simulink model "UAM_GuidanceAndNavigation"  (R2024b)
settings: Solver=FixedStepAuto  StartTime=0.0  StopTime=10.0  RelTol=1e-3
undefined symbols (not defined in the file): Earth, WGS84
libraries: simulink x2, robotcorelib x2, uavalgslib x1, mspfiltlib x1, simulink_extras x1, aerolibtransform2 x1
settings Model: DataDictionary=UAM_data.sldd  Creator=admin  LastModifiedBy=admin
settings OptimizationCC: DefaultParameterBehavior=Inlined  EnhancedBackFolding=on  PassReuseOutputArgsAs=Individual arguments  ZeroExternalMemoryAtStartup=off  ZeroInternalMemoryAtStartup=off  OptimizeBlockOrder=speed  DifferentSizesBufferReuse=on  OptimizationCustomize=off  EfficientTunableParamExpr=on
settings DebuggingCC: ParameterTunabilityLossMsg=error
settings HardwareCC: ProdBitPerLong=64  ProdLargestAtomicInteger=LongLong  ProdLargestAtomicFloat=Double  ProdLongLongMode=on  ProdHWDeviceType=ARM Compatible->ARM Cortex-A (64-bit)
settings SFSimCC: MATLABDynamicMemAlloc=off
settings RTWCC: Description=Embedded Coder  SystemTargetFile=ert.tlc  TemplateMakefile=ert_default_tmf  Toolchain=Linaro AArch64 Linux v6.3.1
settings CodeAppCC: ForceParamTrailComments=on  IgnoreCustomStorageClasses=off  OperatorAnnotations=on  SimulinkDataObjDesc=on  SFDataObjDesc=on  CustomSymbolStrGlobalVar=GUID_$N$M  CustomSymbolStrType=GUID_$N$M_T  CustomSymbolStrField=GUID_$N$M  CustomSymbolStrFcn=GUID_$N$M$F  CustomSymbolStrBlkIO=GUID_rtb_$N$M  CustomSymbolStrTmpVar=GUID_tmp_$N$M  CustomSymbolStrMacro=GUID_$N$M_MACRO  InsertBlockDesc=on
settings ERTTargetCC: TargetLangStandard=C99 (ISO)  GenerateSampleERTMain=on  ERTCustomFileTemplate=example_file_process.tlc

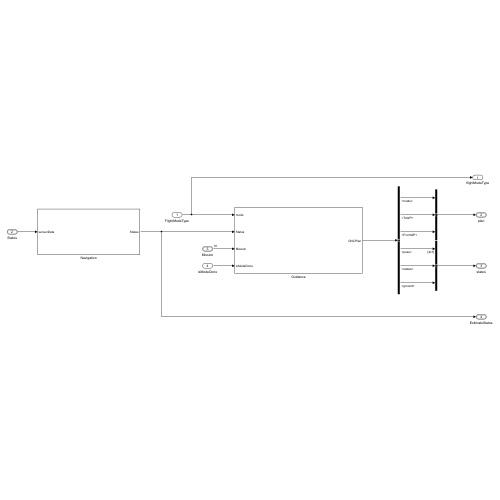
[thumbnail: Simulink's stored preview of the top-level diagram]
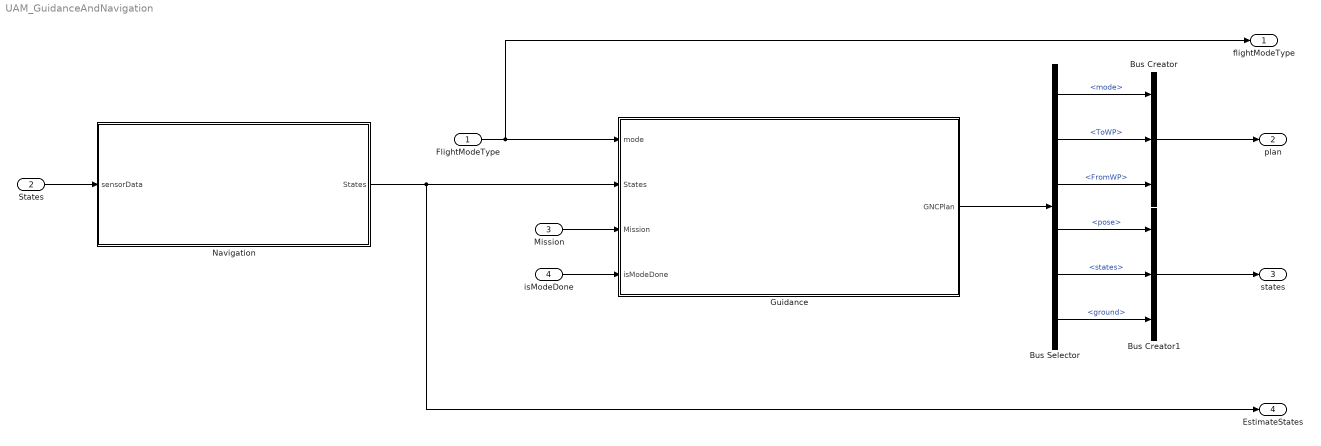
== system UAM_GuidanceAndNavigation ==
  FlightModeType : Inport  OutDataTypeStr=Enum: FlightModeType
  States : Inport  Port=2  OutDataTypeStr=Bus: sensorData
  Mission : Inport  Port=3  OutDataTypeStr=Bus: UAVPathManagerBus  PortDimensions=10  BusOutputAsStruct=on
  isModeDone : Inport  Port=4  OutDataTypeStr=uint8
  Bus Creator : BusCreator  Inputs=3  OutDataTypeStr=Bus: plan
      settings: InheritFromInputs=off
  Bus Creator1 : BusCreator  Inputs=3  OutDataTypeStr=Bus: states
      settings: InheritFromInputs=off
  Bus Selector : BusSelector  OutputSignals=mode,ToWP,FromWP,pose,states,ground
  Guidance : Subsystem
  Navigation : Subsystem
  flightModeType : Outport
  plan : Outport  Port=2  OutDataTypeStr=Bus: plan
  states : Outport  Port=3  OutDataTypeStr=Bus: states
  EstimateStates : Outport  Port=4  OutDataTypeStr=Bus: StateBus
  wires:
  Navigation/1(States) -> EstimateStates/1, Guidance/2(States)
  States/1 -> Navigation/1(sensorData)
  isModeDone/1 -> Guidance/4(isModeDone)
  FlightModeType/1 -> Guidance/1(mode), flightModeType/1
  Bus Creator1/1 -> states/1
  Bus Creator/1 -> plan/1
  Guidance/1(GNCPlan) -> Bus Selector/1
  Bus Selector/1 -> Bus Creator/1  "<mode>"
  Bus Selector/3 -> Bus Creator/3  "<FromWP>"
  Bus Selector/4 -> Bus Creator1/1  "<pose>"
  Bus Selector/5 -> Bus Creator1/2  "<states>"
  Bus Selector/6 -> Bus Creator1/3  "<ground>"
  Bus Selector/2 -> Bus Creator/2  "<ToWP>"
  Mission/1 -> Guidance/3(Mission)

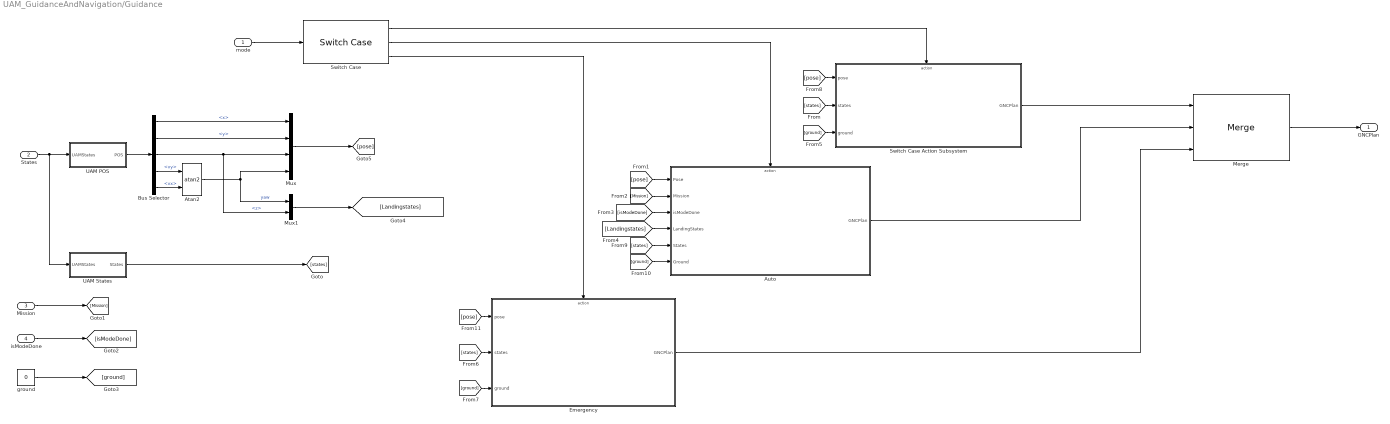
== system UAM_GuidanceAndNavigation/Guidance ==
  mode : Inport
  States : Inport  Port=2
  Mission : Inport  Port=3  OutDataTypeStr=Bus: UAVPathManagerBus
  isModeDone : Inport  Port=4
  Atan2 : Trigonometry  Operator=atan2
  Auto : Subsystem  TreatAsAtomicUnit=on
  Bus Selector : BusSelector  OutputSignals=x,y,z,vy,vx
  Emergency : Subsystem  TreatAsAtomicUnit=on
  Merge : Merge  Inputs=3
  Mux : Mux
  Mux1 : Mux  Inputs=2
  Switch Case : SwitchCase  CaseConditions={FlightModeType.Manual, FlightModeType.Auto, FlightModeType.Emergecny}  ShowDefaultCase=off
  Switch Case Action Subsystem : Subsystem  TreatAsAtomicUnit=on
  UAM POS : Subsystem
  UAM States : Subsystem
  ground : Constant  Value=0
  GNCPlan : Outport  OutDataTypeStr=Bus: GNCplan
  wires:
  mode/1 -> Switch Case/1
  [pose] -> Emergency/1(pose)
  UAM POS/1(POS) -> Bus Selector/1
  [ground] -> Auto/6(Ground)
  [states] -> Switch Case Action Subsystem/2(states)
  Bus Selector/1 -> Mux/1  "<x>"
  Mission/1 -> [Mission]
  [pose] -> Auto/1(Pose)
  [states] -> Emergency/2(states)
  [isModeDone] -> Auto/3(isModeDone)
  Emergency/1(GNCPlan) -> Merge/3
  [ground] -> Switch Case Action Subsystem/3(ground)
  Auto/1(GNCPlan) -> Merge/2
  [ground] -> Emergency/3(ground)
  Switch Case/1 -> Switch Case Action Subsystem/Action
  Bus Selector/2 -> Mux/2  "<y>"
  [Mission] -> Auto/2(Mission)
  Switch Case Action Subsystem/1(GNCPlan) -> Merge/1
  Atan2/1 -> Mux1/1, Mux/4  "yaw"
  ground/1 -> [ground]
  Mux/1 -> [pose]
  Merge/1 -> GNCPlan/1
  Switch Case/3 -> Emergency/Action
  [Landingstates] -> Auto/4(LandingStates)
  isModeDone/1 -> [isModeDone]
  [states] -> Auto/5(States)
  Bus Selector/3 -> Mux1/2, Mux/3  "<z>"
  UAM States/1(States) -> [states]
  [pose] -> Switch Case Action Subsystem/1(pose)
  Switch Case/2 -> Auto/Action
  Mux1/1 -> [Landingstates]
  States/1 -> UAM States/1(UAMStates), UAM POS/1(UAMStates)
  Bus Selector/4 -> Atan2/1  "<vy>"
  Bus Selector/5 -> Atan2/2  "<vx>"

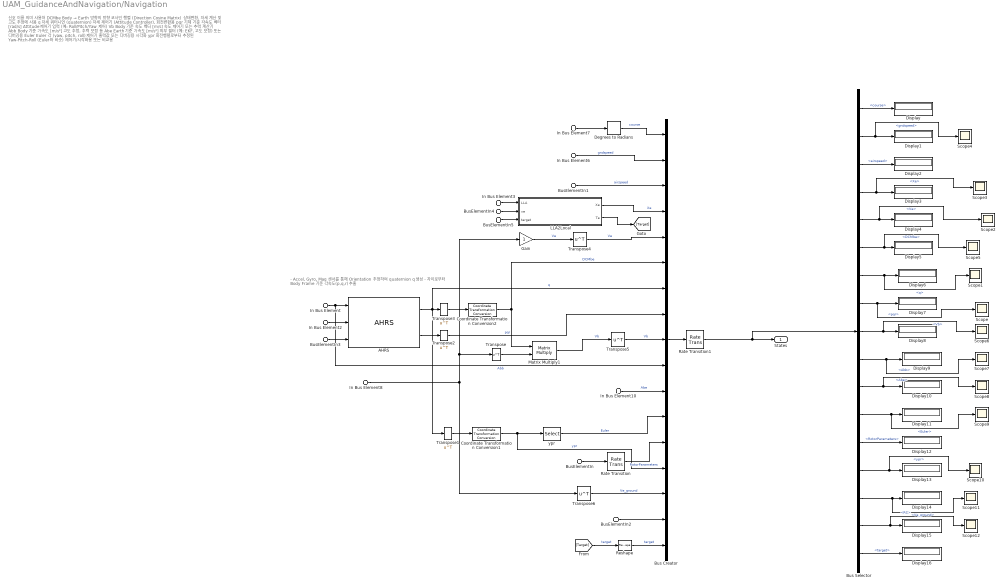
== system UAM_GuidanceAndNavigation/Navigation ==
  note: 신호 이름
      | 의미
      | 사용처
      |
      | DCMbe
      | Body → Earth 방향의 방향 코사인 행렬 (Direction Cosine Matrix)
      | 상태변환, 자세 계산 및 고도 추정에 사용
      |
      | q
      | 자세 쿼터니언 (quaternion)
      | 자세 제어기 (Attitude Controller), 회전변환용
      |
      | pqr
      | 기체 기준 각속도 벡터 [rad/s]
      | Attitude 제어기 입력 (예: Roll/Pitch/Yaw 제어)
      |
      | Vb
      | Body 기준 속도 벡터 [m/s]
      | 속도 제어기 또는 추력 계산기
      |
      | Abb
      | Body 기준 가속도 [m/s²]
      | 고도 추정, 추력 보정 등
      |
      | Abe
      | Earth 기준 가속도 [m/s²]
      | 외부 필터 (예: EKF, 고도 보정) 또는 디버깅용
      |
      | Euler
      | Euler 각 (yaw, pitch, roll)
      | 제어기 출력값 또는 디버깅용 시각화
      |
      | ypr
      | 회전행렬로부터 추정된 Yaw-Pitch-Roll (Euler와 비슷)
      | 제어기/시각화용 또는 비교용
  note: - Accel, Gyro, Mag 센서를 통해 Orientation 추정하여 quaternion q 생성
      | - 자이로부터 Body Frame 기준 각속도(p,q,r) 추출
  In Bus Element : Inport  PortName=sensorData  Element=Abb
  In Bus Element2 : Inport  PortName=sensorData  Element=Gyro
  In Bus Element3 : Inport  PortName=sensorData  Element=LLA
  In Bus Element6 : Inport  PortName=sensorData  Element=gndspeed
  In Bus Element7 : Inport  PortName=sensorData  Element=GPSCourse
  In Bus Element8 : Inport  PortName=sensorData  Element=GPSVelocity
  In Bus Element10 : Inport  PortName=sensorData  Element=Abe
  BusElementIn : Inport  PortName=sensorData  Element=RotorParameters
  BusElementIn1 : Inport  PortName=sensorData  Element=airspeed
  BusElementIn2 : Inport  PortName=sensorData  Element=RC
  BusElementIn5 : Inport  PortName=sensorData  Element=target
  BusElementIn3 : Inport  PortName=sensorData  Element=Mag
  BusElementIn4 : Inport  PortName=sensorData  Element=arming
  AHRS : mspfiltlib/AHRS  DispRefFrame=NED  DecimationFactor=1  InitialProcessNoise=ahrsfilter.defaultProcessNoise  OrientationFormat=quaternion  SimulateUsing=Interpreted execution  AccelerometerNoise=0.0001924722  GyroscopeNoise=9.1385e-5  MagnetometerNoise=0.1  GyroscopeDriftNoise=3.0462e-13  LinearAccelerationNoise=0.0096236100000000012  MagneticDisturbanceNoise=0.5  LinearAccelerationDecayFactor=0.5  MagneticDisturbanceDecayFactor=0.5  ExpectedMagneticFieldStrength=50
  Bus Creator : BusCreator  Inputs=17  OutDataTypeStr=Bus: StateBus
  Bus Selector : BusSelector  OutputSignals=course,gndspeed,airspeed,Xe,Ve,DCMbe,q,pqr,Vb,Abb,Abe,Euler,RotorParameters,ypr,Ve_ground,RC,target
  Coordinate Transformation Conversion1 : robotcorelib/Coordinate Transformation Conversion  InputRepresentation=Quaternion  InputEulerSequence=ZYX  ShowTrVecInputPort=on  OutputRepresentation=Euler Angles  OutputEulerSequence=ZYX  ShowTrVecOutputPort=on  SimulateUsing=Interpreted execution
  Coordinate Transformation Conversion2 : robotcorelib/Coordinate Transformation Conversion  InputRepresentation=Quaternion  InputEulerSequence=ZYX  ShowTrVecInputPort=on  OutputRepresentation=Rotation Matrix  OutputEulerSequence=ZYX  ShowTrVecOutputPort=on  SimulateUsing=Interpreted execution
  Degrees to Radians : simulink_extras/Transformations/Degrees to Radians
  Display{,1..16} (17 alike) : Display
  Gain : Gain
  LLA2Local : Subsystem
  Matrix Multiply1 : Product  Multiplication=Matrix(*)
  Rate Transition : RateTransition  OutPortSampleTime=0.001
  Rate Transition1 : RateTransition
  Reshape : Reshape  OutputDimensionality=Customize  OutputDimensions=[1 3]
  Scope{,1..12} (13 alike) : Scope
  Transpose{,1..6} (7 alike) : Math  Operator=transpose
  ypr : Selector  InputPortWidth=3  IndexOptions=Index vector (dialog)  Indices=[3 2 1]  OutputSizes=1
  States : Outport  OutDataTypeStr=Bus: StateBus
  wires:
  Transpose6/1 -> Bus Creator/15  "Ve_ground"
  In Bus Element/1 -> AHRS/1, Bus Creator/10  "Abb"
  ypr/1 -> Bus Creator/12  "Euler"
  Gain/1 -> Transpose4/1  "Ve"
  Transpose/1 -> Matrix Multiply1/2
  LLA2Local/1(Xe) -> Bus Creator/4  "Xe"
  Matrix Multiply1/1 -> Transpose5/1  "Vb"
  In Bus Element8/1 -> Gain/1, Transpose/1, Transpose6/1
  In Bus Element7/1 -> Degrees to Radians/1
  Rate Transition1/1 -> Bus Selector/1, States/1
  In Bus Element6/1 -> Bus Creator/2  "gndspeed"
  Coordinate Transformation Conversion2/1 -> Bus Creator/6, Matrix Multiply1/1  "DCMbe"
  Transpose5/1 -> Bus Creator/9  "Vb"
  Transpose2/1 -> Bus Creator/8  "pqr"
  Coordinate Transformation Conversion1/1 -> Bus Creator/14, ypr/1  "ypr"
  In Bus Element10/1 -> Bus Creator/11  "Abe"
  Bus Creator/1 -> Rate Transition1/1
  Rate Transition/1 -> Bus Creator/13  "RotorParameters"
  Degrees to Radians/1 -> Bus Creator/1  "course"
  Transpose4/1 -> Bus Creator/5  "Ve"
  In Bus Element3/1 -> LLA2Local/1(LLA)
  BusElementIn/1 -> Rate Transition/1
  BusElementIn1/1 -> Bus Creator/3  "airspeed"
  BusElementIn2/1 -> Bus Creator/16
  Transpose1/1 -> Coordinate Transformation Conversion1/1
  Transpose3/1 -> Coordinate Transformation Conversion2/1
  LLA2Local/2(Te) -> [Target]
  [Target] -> Reshape/1  "target"
  BusElementIn5/1 -> LLA2Local/3(target)
  Reshape/1 -> Bus Creator/17  "target"
  In Bus Element2/1 -> AHRS/2
  BusElementIn3/1 -> AHRS/3
  AHRS/1 -> Transpose3/1, Transpose1/1, Bus Creator/7  "q"
  AHRS/2 -> Transpose2/1
  BusElementIn4/1 -> LLA2Local/2(ve)
  Bus Selector/1 -> Display/1  "<course>"
  Bus Selector/2 -> Scope4/1, Display1/1  "<gndspeed>"
  Bus Selector/3 -> Display2/1  "<airspeed>"
  Bus Selector/4 -> Scope3/1, Display3/1  "<Xe>"
  Bus Selector/5 -> Scope2/1, Display4/1  "<Ve>"
  Bus Selector/6 -> Scope5/1, Display5/1  "<DCMbe>"
  Bus Selector/7 -> Scope1/1, Display6/1  "<q>"
  Bus Selector/8 -> Scope/1, Display7/1  "<pqr>"
  Bus Selector/9 -> Scope6/1, Display8/1  "<Vb>"
  Bus Selector/10 -> Scope7/1, Display9/1  "<Abb>"
  Bus Selector/11 -> Scope8/1, Display10/1  "<Abe>"
  Bus Selector/12 -> Scope9/1, Display11/1  "<Euler>"
  Bus Selector/13 -> Display12/1  "<RotorParameters>"
  Bus Selector/14 -> Scope10/1, Display13/1  "<ypr>"
  Bus Selector/15 -> Scope11/1, Display14/1  "<Ve_ground>"
  Bus Selector/16 -> Scope12/1, Display15/1  "<RC>"
  Bus Selector/17 -> Display16/1  "<target>"

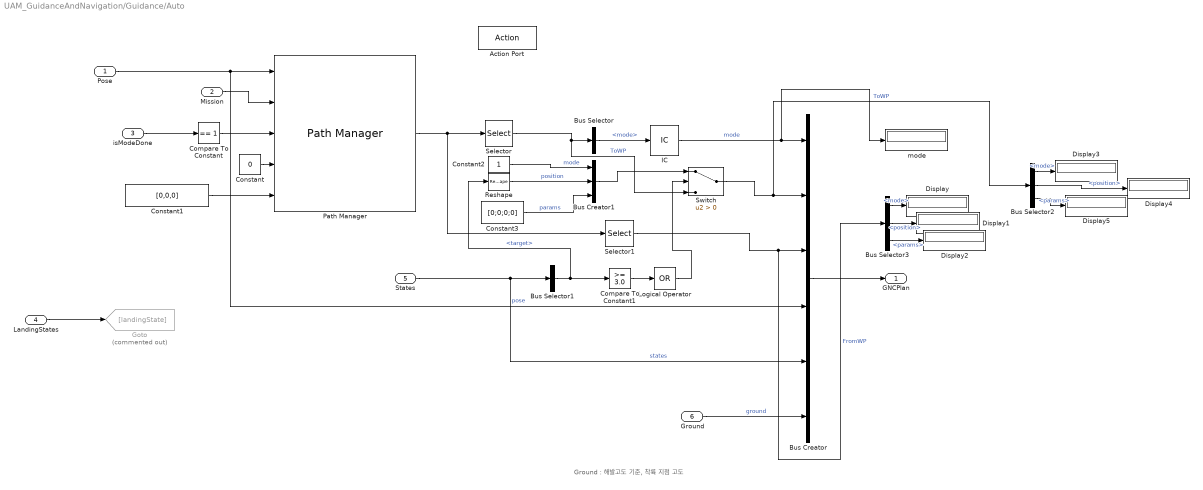
== system UAM_GuidanceAndNavigation/Guidance/Auto ==
  note: Ground : 해발고도 기준, 착륙 지점 고도
  Pose : Inport
  Mission : Inport  Port=2  OutDataTypeStr=Bus: UAVPathManagerBus
  isModeDone : Inport  Port=3
  LandingStates : Inport  Port=4
  States : Inport  Port=5
  Ground : Inport  Port=6
  Action Port : ActionPort  ActionPortLabel=case [ Auto ]:
  Bus Creator : BusCreator  Inputs=6  OutDataTypeStr=Bus: GNCplan
  Bus Creator1 : BusCreator  Inputs=3  OutDataTypeStr=Bus: UAVPathManagerBus  NonVirtualBus=on
  Bus Selector : BusSelector  OutputSignals=mode
  Bus Selector1 : BusSelector  OutputSignals=target
  Bus Selector2 : BusSelector  OutputSignals=mode,position,params
  Bus Selector3 : BusSelector  OutputSignals=mode,position,params
  Compare To Constant : simulink/Logic and Bit Operations/Compare To Constant  relop===  const=1  OutDataTypeStr=boolean
  Compare To Constant1 : simulink/Logic and Bit Operations/Compare To Constant  relop=>=  const=3.0  OutDataTypeStr=boolean
  Constant : Constant  Value=0  OutDataTypeStr=uint8
  Constant1 : Constant  Value=[0,0,0]  OutDataTypeStr=double
  Constant2 : Constant  OutDataTypeStr=uint8
  Constant3 : Constant  Value=[0;0;0;0]
  Display{,1..5} (6 alike) : Display
  Goto : Goto  Commented=on  GotoTag=landingState
  IC : InitialCondition
  Logical Operator : Logic  Operator=OR  Inputs=1  AllPortsSameDT=off  OutDataTypeStr=boolean
  Path Manager : uavalgslib/Path Manager  UAVType=multirotor  LoiterRadius=25  dataType=double  inputBusName='UAVPathManagerBus'  SimulateUsing=Code generation
  Reshape : Reshape  OutputDimensionality=Customize  OutputDimensions=[3 1]
  Selector : Selector  InputPortWidth=2  IndexOptions=Index vector (dialog)  Indices=1  OutputSizes=1
  Selector1 : Selector  InputPortWidth=2  IndexOptions=Index vector (dialog)  Indices=2  OutputSizes=1
  Switch : Switch  Criteria=u2 > Threshold  SaturateOnIntegerOverflow=off  InputSameDT=off
  mode : Display
  GNCPlan : Outport  OutDataTypeStr=Bus: GNCplan
  wires:
  IC/1 -> mode/1, Bus Creator/1  "mode"
  Ground/1 -> Bus Creator/6  "ground"
  Selector1/1 -> Bus Selector3/1, Bus Creator/3  "FromWP"
  States/1 -> Bus Selector1/1, Bus Creator/5  "states"
  Bus Creator/1 -> GNCPlan/1
  Selector/1 -> Bus Selector/1, Switch/3  "ToWP"
  Path Manager/1 -> Selector/1, Selector1/1
  Constant/1 -> Path Manager/4
  Constant1/1 -> Path Manager/5
  Pose/1 -> Bus Creator/4, Path Manager/1  "pose"
  LandingStates/1 -> Goto/1
  Compare To Constant/1 -> Path Manager/3
  isModeDone/1 -> Compare To Constant/1
  Bus Selector/1 -> IC/1  "<mode>"
  Mission/1 -> Path Manager/2
  Bus Selector1/1 -> Reshape/1, Compare To Constant1/1  "<target>"
  Compare To Constant1/1 -> Logical Operator/1
  Logical Operator/1 -> Switch/2
  Switch/1 -> Bus Selector2/1, Bus Creator/2  "ToWP"
  Constant2/1 -> Bus Creator1/1  "mode"
  Constant3/1 -> Bus Creator1/3  "params"
  Reshape/1 -> Bus Creator1/2  "position"
  Bus Creator1/1 -> Switch/1
  Bus Selector3/1 -> Display/1  "<mode>"
  Bus Selector3/2 -> Display1/1  "<position>"
  Bus Selector3/3 -> Display2/1  "<params>"
  Bus Selector2/1 -> Display3/1  "<mode>"
  Bus Selector2/2 -> Display4/1  "<position>"
  Bus Selector2/3 -> Display5/1  "<params>"

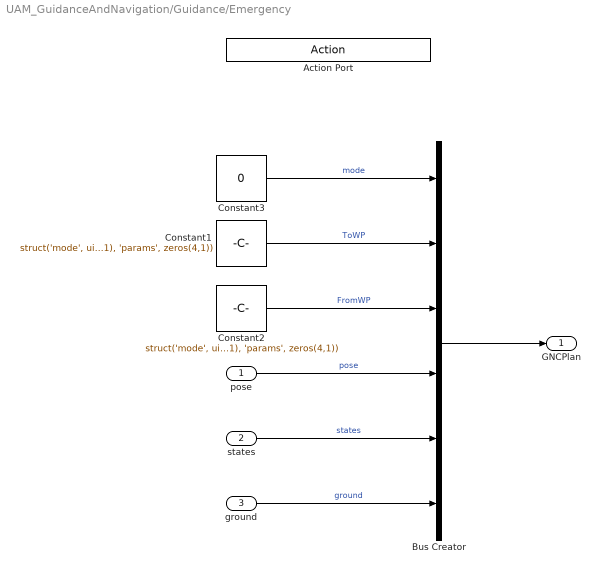
== system UAM_GuidanceAndNavigation/Guidance/Emergency ==
  pose : Inport
  states : Inport  Port=2
  ground : Inport  Port=3
  Action Port : ActionPort  ActionPortLabel=case [ Emergecny ]:
  Bus Creator : BusCreator  Inputs=6  OutDataTypeStr=Bus: GNCplan
  Constant1 : Constant  Value=struct('mode', uint8(0), 'position', zeros(3,1), 'params', zeros(4,1))  OutDataTypeStr=Bus: UAVPathManagerBus
  Constant2 : Constant  Value=struct('mode', uint8(0), 'position', zeros(3,1), 'params', zeros(4,1))  OutDataTypeStr=Bus: UAVPathManagerBus
  Constant3 : Constant  Value=0  OutDataTypeStr=uint8
  GNCPlan : Outport  OutDataTypeStr=Bus: GNCplan
  wires:
  pose/1 -> Bus Creator/4  "pose"
  Bus Creator/1 -> GNCPlan/1
  Constant1/1 -> Bus Creator/2  "ToWP"
  Constant2/1 -> Bus Creator/3  "FromWP"
  ground/1 -> Bus Creator/6  "ground"
  states/1 -> Bus Creator/5  "states"
  Constant3/1 -> Bus Creator/1  "mode"

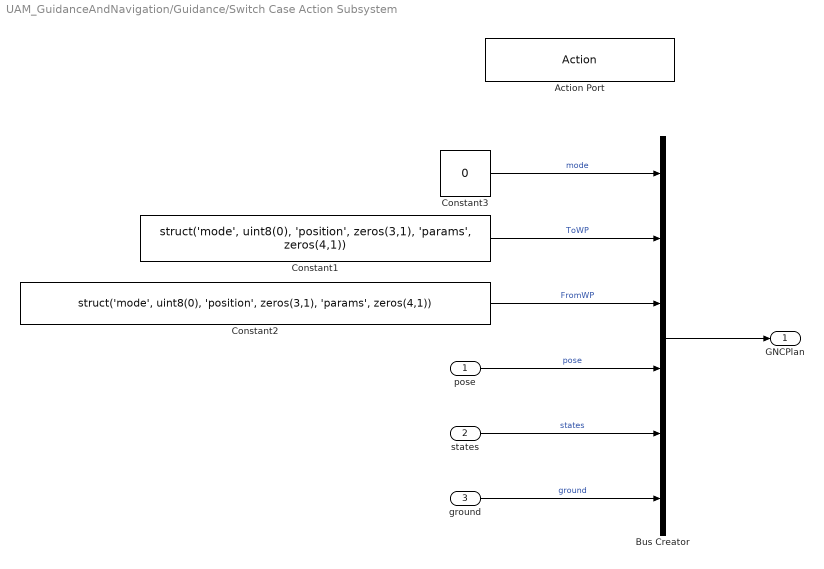
== system UAM_GuidanceAndNavigation/Guidance/Switch Case Action Subsystem ==
  pose : Inport
  states : Inport  Port=2
  ground : Inport  Port=3
  Action Port : ActionPort  ActionPortLabel=case [ Manual ]:
  Bus Creator : BusCreator  Inputs=6  OutDataTypeStr=Bus: GNCplan
  Constant1 : Constant  Value=struct('mode', uint8(0), 'position', zeros(3,1), 'params', zeros(4,1))  OutDataTypeStr=Bus: UAVPathManagerBus
  Constant2 : Constant  Value=struct('mode', uint8(0), 'position', zeros(3,1), 'params', zeros(4,1))  OutDataTypeStr=Bus: UAVPathManagerBus
  Constant3 : Constant  Value=0  OutDataTypeStr=uint8
  GNCPlan : Outport  OutDataTypeStr=Bus: GNCplan
  wires:
  Bus Creator/1 -> GNCPlan/1
  Constant3/1 -> Bus Creator/1  "mode"
  Constant2/1 -> Bus Creator/3  "FromWP"
  Constant1/1 -> Bus Creator/2  "ToWP"
  pose/1 -> Bus Creator/4  "pose"
  states/1 -> Bus Creator/5  "states"
  ground/1 -> Bus Creator/6  "ground"

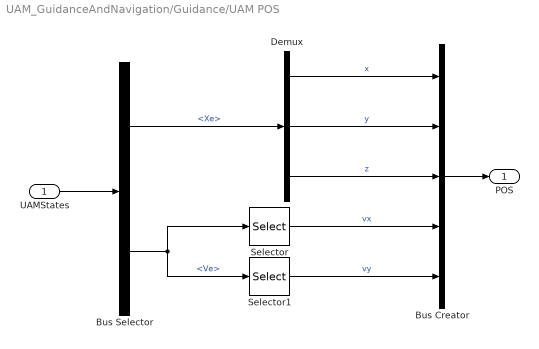
== system UAM_GuidanceAndNavigation/Guidance/UAM POS ==
  UAMStates : Inport  OutDataTypeStr=Bus: StateBus
  Bus Creator : BusCreator  Inputs=5
  Bus Selector : BusSelector  OutputSignals=Xe,Ve
  Demux : Demux  Outputs=3
  Selector : Selector  InputPortWidth=3  IndexOptions=Index vector (dialog)  Indices=[1]  OutputSizes=1
  Selector1 : Selector  InputPortWidth=3  IndexOptions=Index vector (dialog)  Indices=[2]  OutputSizes=1
  POS : Outport
  wires:
  UAMStates/1 -> Bus Selector/1
  Bus Selector/1 -> Demux/1  "<Xe>"
  Demux/1 -> Bus Creator/1  "x"
  Demux/2 -> Bus Creator/2  "y"
  Demux/3 -> Bus Creator/3  "z"
  Bus Selector/2 -> Selector/1, Selector1/1  "<Ve>"
  Selector/1 -> Bus Creator/4  "vx"
  Selector1/1 -> Bus Creator/5  "vy"
  Bus Creator/1 -> POS/1

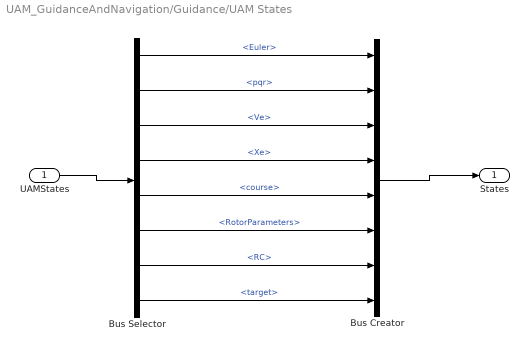
== system UAM_GuidanceAndNavigation/Guidance/UAM States ==
  UAMStates : Inport
  Bus Creator : BusCreator  Inputs=8
  Bus Selector : BusSelector  OutputSignals=Euler,pqr,Ve,Xe,course,RotorParameters,RC,target
  States : Outport
  wires:
  UAMStates/1 -> Bus Selector/1
  Bus Selector/3 -> Bus Creator/3  "<Ve>"
  Bus Selector/1 -> Bus Creator/1  "<Euler>"
  Bus Selector/2 -> Bus Creator/2  "<pqr>"
  Bus Selector/4 -> Bus Creator/4  "<Xe>"
  Bus Selector/5 -> Bus Creator/5  "<course>"
  Bus Selector/6 -> Bus Creator/6  "<RotorParameters>"
  Bus Creator/1 -> States/1
  Bus Selector/7 -> Bus Creator/7  "<RC>"
  Bus Selector/8 -> Bus Creator/8  "<target>"

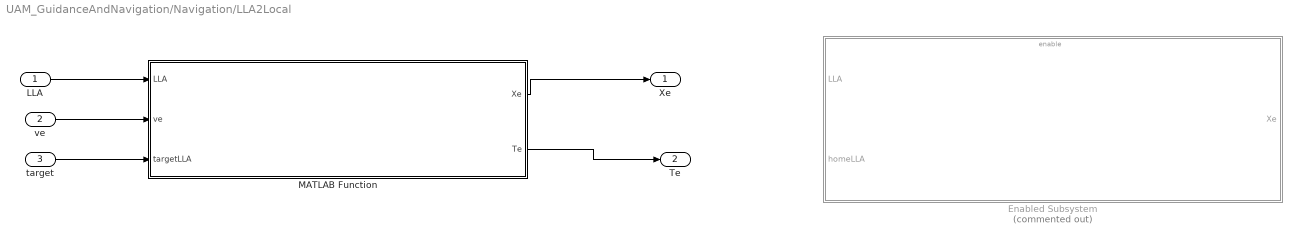
== system UAM_GuidanceAndNavigation/Navigation/LLA2Local ==
  LLA : Inport
  ve : Inport  Port=2
  target : Inport  Port=3
  Enabled Subsystem : Subsystem  Commented=on  TreatAsAtomicUnit=on
  MATLAB Function : MATLAB Function  TreatAsAtomicUnit=on
  Xe : Outport
  Te : Outport  Port=2
  wires:
  LLA/1 -> MATLAB Function/1(LLA)
  ve/1 -> MATLAB Function/2(ve)
  MATLAB Function/1(Xe) -> Xe/1
  MATLAB Function/2(Te) -> Te/1
  target/1 -> MATLAB Function/3(targetLLA)

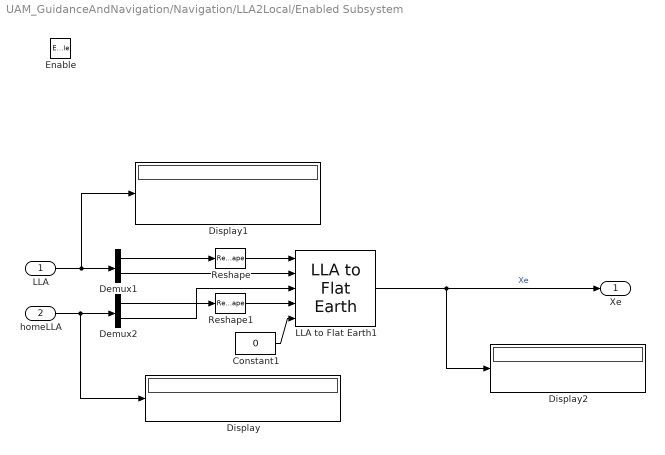
== system UAM_GuidanceAndNavigation/Navigation/LLA2Local/Enabled Subsystem ==
  LLA : Inport
  homeLLA : Inport  Port=2
  Enable : EnablePort
  Constant1 : Constant  Value=0
  Demux1 : Demux  Outputs=[2 1]
  Demux2 : Demux  Outputs=[2 1]
  Display : Display
  Display1 : Display
  Display2 : Display
  LLA to Flat Earth1 : aerolibtransform2/LLA to Flat Earth  units=Metric (MKS)  ptype=Earth (WGS84)  F=1/298.257223563  R=6378137  refPosPort=on  LL0=[0,0]  psi=0
  Reshape : Reshape  OutputDimensionality=Customize  OutputDimensions=[2 1]
  Reshape1 : Reshape  OutputDimensionality=Customize  OutputDimensions=[2 1]
  Xe : Outport
  wires:
  Constant1/1 -> LLA to Flat Earth1/5
  LLA to Flat Earth1/1 -> Display2/1, Xe/1  "Xe"
  Demux1/2 -> LLA to Flat Earth1/2
  Demux1/1 -> Reshape/1
  homeLLA/1 -> Display/1, Demux2/1
  LLA/1 -> Display1/1, Demux1/1
  Demux2/2 -> LLA to Flat Earth1/3
  Demux2/1 -> Reshape1/1
  Reshape/1 -> LLA to Flat Earth1/1
  Reshape1/1 -> LLA to Flat Earth1/4

== matlab function UAM_GuidanceAndNavigation/Navigation/LLA2Local/MATLAB Function ==
  data: LLA input; Xe output; ve input; targetLLA input; Te output
function [Xe, Te] = NEDfromLLA_withTarget(LLA, ve, targetLLA)
%#codegen
% 입력
%   LLA       : [1x3] 현재 [lat, lon, alt] (deg,deg,m)
%   ve        : [1x3] 현재 속도 [vx,vy,vz] (m/s) - 홈 설정(정지판정)용
%   targetLLA : [1x3] 타깃 [lat, lon, alt] (deg,deg,m)
%
% 출력
%   Xe : [3x1] 현재 위치 NED (Home 기준)
%   Te : [3x1] 타깃 위치 NED (Home 기준)

    persistent isSet homeLLA
    if isempty(isSet)
        isSet   = false;
        homeLLA = [NaN, NaN, NaN];
    end

    % 홈포인트 1회 설정 (정지 + 유효 LLA)
    speed = norm(ve);
    if ~isSet && speed < 0.5 && all(isfinite(LLA)) && any(LLA ~= 0)
        homeLLA = LLA;
        isSet   = true;
    end

    % 홈 미설정이면 0 리턴
    if ~isSet
        Xe = zeros(3,1);
        Te = zeros(3,1);
        return;
    end

    % 현재/타깃 LLA → NED (같은 Home 기준)
    Xe = lla2ned_local(LLA, homeLLA);

    if all(isfinite(targetLLA)) && any(targetLLA ~= 0)
        Te = lla2ned_local(targetLLA, homeLLA);
    else
        Te = zeros(3,1);
    end
end

% --- 지역함수: 소범위 LLA→NED 근사 ---
function ned = lla2ned_local(LLA, homeLLA)
    a  = 6378137.0;                  % WGS-84 semi-major axis
    f  = 1/298.257223563;            % flattening
    e2 = f*(2 - f);

    lat0 = deg2rad(homeLLA(1));
    dLat = deg2rad(LLA(1) - homeLLA(1));
    dLon = deg2rad(LLA(2) - homeLLA(2));
    dAlt = (LLA(3) - homeLLA(3));

    sin0 = sin(lat0); cos0 = cos(lat0);
    RN = a / sqrt(1 - e2*sin0*sin0);
    RM = RN * (1 - e2) / (1 - e2*sin0*sin0);

    dN = RM * dLat;           % North (m)
    dE = RN * cos0 * dLon;    % East  (m)
    dD = -dAlt;               % Down  (m)

    ned = [dN; dE; dD];       % 3x1
end
